simulink model "sampling_give_new_frequencies"  (R2018b)
settings: Solver=VariableStepAuto  StartTime=0.0  StopTime=18  RelTol=1e-3
model workspace (MATLAB code in the model file):
  | fr = 5.1; % Resonance freq
  | omega_1 = fr*2*pi;
  | zeta_z = 0.1;
  | zeta_p = 0.01;
  | fs = 10; % Sampling freq
  | h = 1.0/fs; % Sampling period
  | fe = 4.9; % Excitation freq
  | omega_e = 2*pi*fe;
  | num = [1, 2*zeta_z*omega_1, omega_1*omega_1];
  | den = [1, 2*zeta_p*omega_1, omega_1*omega_1];
  | G = tf(num, den);
  | figure(1)
  | clf
  | pzmap(G)
  | axis equal
  | 
  | 
  | figure(2)
  | clf
  | bode(G)
settings Model: Creator=kjartan  LastModifiedBy=kjartan
settings SFSimCC: SimUseLocalCustomCode=off
settings RTWCC: RTWUseLocalCustomCode=off
settings CodeAppCC: StateflowObjectComments=on

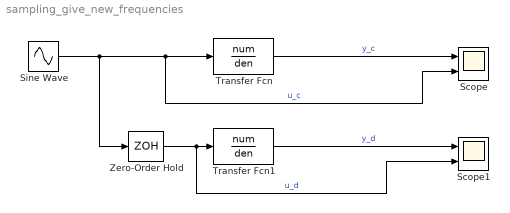
== system sampling_give_new_frequencies ==
  Scope : Scope  NumInputPorts=2
  Scope1 : Scope  NumInputPorts=2
  Sine Wave : Sin  Frequency=3*2*pi  SampleTime=0
  Transfer Fcn : TransferFcn  Numerator=num  Denominator=den
  Transfer Fcn1 : TransferFcn  Numerator=num  Denominator=den
  Zero-Order Hold : ZeroOrderHold  SampleTime=1/8
  wires:
  Sine Wave/1 -> Zero-Order Hold/1, Scope/2, Transfer Fcn/1  "u_c"
  Zero-Order Hold/1 -> Scope1/2, Transfer Fcn1/1  "u_d"
  Transfer Fcn/1 -> Scope/1  "y_c"
  Transfer Fcn1/1 -> Scope1/1  "y_d"
